simulink model "tcp10"  (R2014a)
settings: Solver=FixedStepDiscrete  StartTime=0.0  StopTime=inf  FixedStep=0.2  RelTol=1e-3
libraries: simulink x6, instrumentlib x4, hdlsllib x2
settings Model: Creator=laca  LastModifiedBy=laca
settings DataIOCC: SignalLoggingSaveFormat=ModelDataLogs

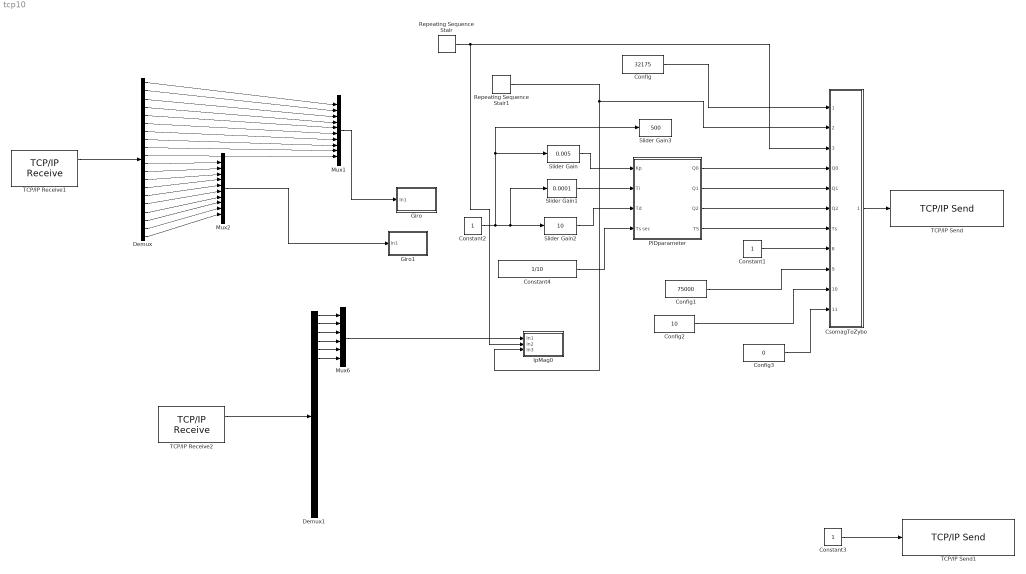
== system tcp10 ==
  Config : Constant  Value=32175
  Config1 : Constant  Value=75000
  Config2 : Constant  Value=10
  Config3 : Constant  Value=0
  Constant1 : Constant
  Constant2 : Constant
  Constant3 : Constant
  Constant4 : Constant  Value=1/10
  CsomagToZybo : Subsystem
  Demux : Demux  Outputs=20
  Demux1 : Demux  Outputs=24
  Giro : Subsystem
  Giro1 : Subsystem
  IpMag0 : Subsystem
  Mux1 : Mux  Inputs=10
  Mux2 : Mux  Inputs=10
  Mux6 : Mux  Inputs=6
  PIDparameter : Subsystem
  Repeating Sequence Stair : simulink/Sources/Repeating Sequence Stair  OutValues=[250*ones(1,1000) 500*ones(1,1000) 800*ones(1,1000) 50*ones(1,1000)].'  tsamp=-1  OutMin=[]  OutMax=[]  OutDataTypeStr=double  OutputDataTypeScalingMode=double  OutDataType=fixdt(0,8)  ConRadixGroup=Best Precision: Vector-wise  OutScaling=2^-12
  Repeating Sequence Stair1 : simulink/Sources/Repeating Sequence Stair  OutValues=[0*ones(1,500) 100*ones(1,500) 77*ones(1,500) -77*ones(1,500) ].'  tsamp=-1  OutMin=[]  OutMax=[]  OutDataTypeStr=double  OutputDataTypeScalingMode=double  OutDataType=fixdt(0,8)  ConRadixGroup=Best Precision: Vector-wise  OutScaling=2^-12
  Slider Gain : simulink/Math Operations/Slider Gain  low=0  gain=0.005  high=65000
  Slider Gain1 : simulink/Math Operations/Slider Gain  low=0  gain=0.0001  high=100000
  Slider Gain2 : simulink/Math Operations/Slider Gain  low=0  gain=10  high=5000
  Slider Gain3 : simulink/Math Operations/Slider Gain  low=-7000  gain=500  high=7000
  TCP/IP Receive1 : instrumentlib/TCP//IP Receive  Host=192.168.0.10  Port=7  DataSize="[1  20]"  EnableBlockingMode=off  Timeout=100  SampleTime=0.2  DataType=int16  ByteOrder=LittleEndian
  TCP/IP Receive2 : instrumentlib/TCP//IP Receive  Host=192.168.0.10  Port=8  DataSize="[1  24]"  EnableBlockingMode=off  Timeout=100  SampleTime=0.2  DataType=int32  ByteOrder=LittleEndian
  TCP/IP Send : instrumentlib/TCP//IP Send  Host=192.168.0.10  Port=7  EnableBlockingMode=off  Timeout=10  ByteOrder=LittleEndian
  TCP/IP Send1 : instrumentlib/TCP//IP Send  Host=192.168.0.10  Port=8  EnableBlockingMode=off  Timeout=10  ByteOrder=LittleEndian
  wires:
  Demux/1 -> Mux1/1
  Demux/2 -> Mux1/2
  Demux/3 -> Mux1/3
  TCP/IP Receive1/1 -> Demux/1
  Mux6/1 -> IpMag0/1(In1)
  Demux/10 -> Mux1/10
  Demux/9 -> Mux1/9
  Demux/8 -> Mux1/8
  Demux/7 -> Mux1/7
  Demux/6 -> Mux1/6
  Demux/5 -> Mux1/5
  Demux/4 -> Mux1/4
  Mux1/1 -> Giro/1(In1)
  CsomagToZybo/1(Out1) -> TCP/IP Send/1
  Constant2/1 -> Slider Gain3/1, Slider Gain/1, Slider Gain1/1, Slider Gain2/1
  Slider Gain/1 -> PIDparameter/1(Kp)
  Slider Gain1/1 -> PIDparameter/2(Ti)
  Slider Gain2/1 -> PIDparameter/3(Td)
  Constant4/1 -> PIDparameter/4(Ts sec)
  PIDparameter/4(TS) -> CsomagToZybo/7(Ts)
  PIDparameter/3(Q2) -> CsomagToZybo/6(Q2)
  PIDparameter/2(Q1) -> CsomagToZybo/5(Q1)
  PIDparameter/1(Q0) -> CsomagToZybo/4(Q0)
  Config/1 -> CsomagToZybo/1(Config)
  Constant1/1 -> CsomagToZybo/8(Egyeb)
  Config1/1 -> CsomagToZybo/9(PwmFrek)
  Config2/1 -> CsomagToZybo/10(qSav)
  Config3/1 -> CsomagToZybo/11(SugaeakAranya)
  Demux/11 -> Mux2/1
  Demux/12 -> Mux2/2
  Demux/13 -> Mux2/3
  Demux/14 -> Mux2/4
  Demux/15 -> Mux2/5
  Demux/16 -> Mux2/6
  Demux/17 -> Mux2/7
  Demux/18 -> Mux2/8
  Demux/19 -> Mux2/9
  Demux/20 -> Mux2/10
  Mux2/1 -> Giro1/1(In1)
  TCP/IP Receive2/1 -> Demux1/1
  Constant3/1 -> TCP/IP Send1/1
  Repeating Sequence Stair/1 -> IpMag0/2(In2), CsomagToZybo/3(RefSpeed)
  Repeating Sequence Stair1/1 -> IpMag0/3(In3), CsomagToZybo/2(RefPos)
  Demux1/6 -> Mux6/6
  Demux1/5 -> Mux6/5
  Demux1/4 -> Mux6/4
  Demux1/3 -> Mux6/3
  Demux1/2 -> Mux6/2
  Demux1/1 -> Mux6/1

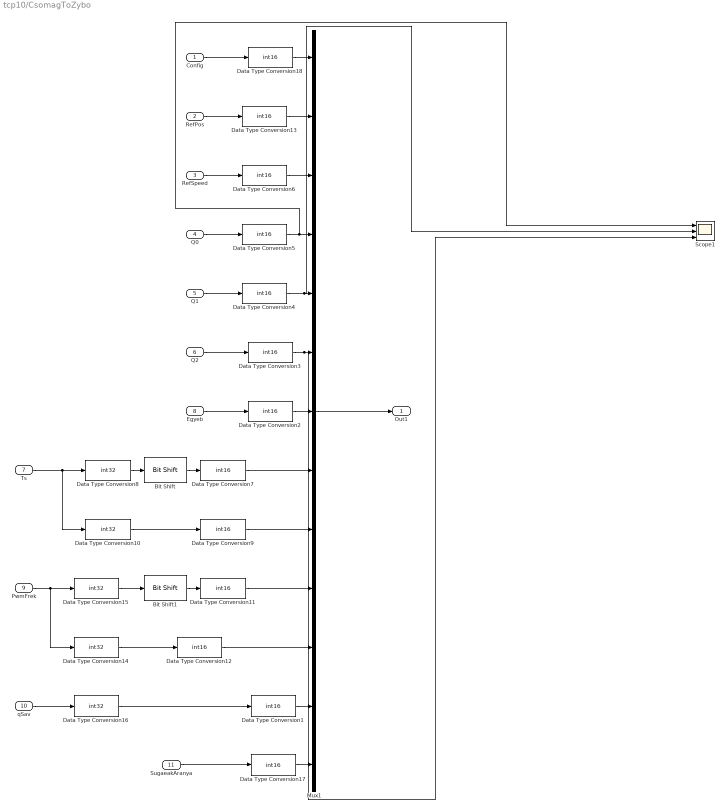
== system tcp10/CsomagToZybo ==
  Config : Inport
  RefPos : Inport  Port=2
  RefSpeed : Inport  Port=3
  Q0 : Inport  Port=4
  Q1 : Inport  Port=5
  Q2 : Inport  Port=6
  Ts : Inport  Port=7
  Egyeb : Inport  Port=8
  PwmFrek : Inport  Port=9
  qSav : Inport  Port=10
  SugaeakAranya : Inport  Port=11
  Bit Shift : hdlsllib/HDL Operations/Bit Shift  mode=Shift Right Arithmetic  N=16
  Bit Shift1 : hdlsllib/HDL Operations/Bit Shift  mode=Shift Right Arithmetic  N=16
  Data Type Conversion{1..7,9,11..13,17..18} (13 alike) : DataTypeConversion  OutDataTypeStr=int16
  Data Type Conversion{8,10,14..16} (5 alike) : DataTypeConversion  OutDataTypeStr=int32
  Mux1 : Mux  Inputs=13
  Scope1 : Scope  NumInputPorts=3
      settings: YMin=1425~-525~-1  YMax=1575~-475~1  SaveName=ScopeData5
  Out1 : Outport
  wires:
  Mux1/1 -> Out1/1
  Data Type Conversion18/1 -> Mux1/1
  Data Type Conversion13/1 -> Mux1/2
  Data Type Conversion6/1 -> Mux1/3
  Data Type Conversion2/1 -> Mux1/7
  Config/1 -> Data Type Conversion18/1
  RefPos/1 -> Data Type Conversion13/1
  RefSpeed/1 -> Data Type Conversion6/1
  Q0/1 -> Data Type Conversion5/1
  Q1/1 -> Data Type Conversion4/1
  Q2/1 -> Data Type Conversion3/1
  Egyeb/1 -> Data Type Conversion2/1
  Ts/1 -> Data Type Conversion10/1, Data Type Conversion8/1
  Data Type Conversion10/1 -> Data Type Conversion9/1
  Data Type Conversion8/1 -> Bit Shift/1
  Bit Shift/1 -> Data Type Conversion7/1
  Data Type Conversion1/1 -> Mux1/12
  PwmFrek/1 -> Data Type Conversion14/1, Data Type Conversion15/1
  Data Type Conversion14/1 -> Data Type Conversion12/1
  Data Type Conversion15/1 -> Bit Shift1/1
  Bit Shift1/1 -> Data Type Conversion11/1
  Data Type Conversion16/1 -> Data Type Conversion1/1
  qSav/1 -> Data Type Conversion16/1
  Data Type Conversion17/1 -> Mux1/13
  SugaeakAranya/1 -> Data Type Conversion17/1
  Data Type Conversion7/1 -> Mux1/8
  Data Type Conversion9/1 -> Mux1/9
  Data Type Conversion11/1 -> Mux1/10
  Data Type Conversion12/1 -> Mux1/11
  Data Type Conversion5/1 -> Scope1/1, Mux1/4
  Data Type Conversion4/1 -> Scope1/2, Mux1/5
  Data Type Conversion3/1 -> Scope1/3, Mux1/6

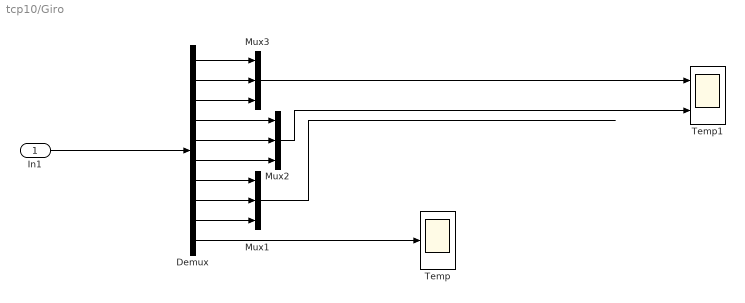
== system tcp10/Giro ==
  In1 : Inport
  Demux : Demux  Outputs=10
  Mux1 : Mux  Inputs=3
  Mux2 : Mux  Inputs=3
  Mux3 : Mux  Inputs=3
  Temp : Scope
      settings: TickLabels=on  TimeRange=2000  YMin=204.25  YMax=225.75  SaveName=ScopeData4  SampleInput=on
  Temp1 : Scope  NumInputPorts=2
      settings: TickLabels=on  TimeRange=250  YMin=-35000~-35000  YMax=35000~35000  SaveName=ScopeData2  SampleInput=on
  wires:
  In1/1 -> Demux/1
  Demux/1 -> Mux3/1
  Demux/2 -> Mux3/2
  Demux/3 -> Mux3/3
  Demux/4 -> Mux2/1
  Demux/5 -> Mux2/2
  Demux/6 -> Mux2/3
  Demux/7 -> Mux1/1
  Demux/8 -> Mux1/2
  Demux/9 -> Mux1/3
  Mux3/1 -> Temp1/1
  Mux2/1 -> Temp1/2
  Mux1/1 -> ?
  Demux/10 -> Temp/1

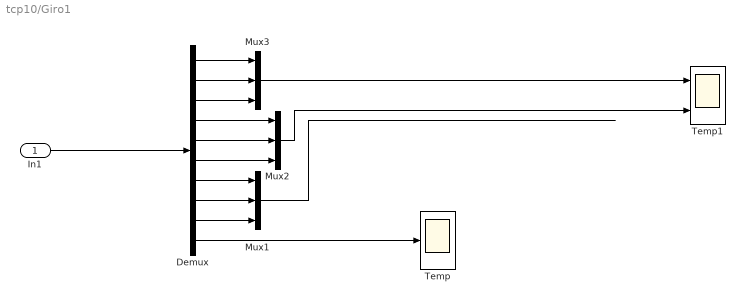
== system tcp10/Giro1 ==
  In1 : Inport
  Demux : Demux  Outputs=10
  Mux1 : Mux  Inputs=3
  Mux2 : Mux  Inputs=3
  Mux3 : Mux  Inputs=3
  Temp : Scope
      settings: TickLabels=on  TimeRange=2000  YMin=36  YMax=36  SaveName=ScopeData4  SampleInput=on
  Temp1 : Scope  NumInputPorts=2
      settings: TickLabels=on  TimeRange=250  YMin=-65500~-35000  YMax=65500~35000  SaveName=ScopeData2  SampleInput=on
  wires:
  In1/1 -> Demux/1
  Demux/1 -> Mux3/1
  Demux/2 -> Mux3/2
  Demux/3 -> Mux3/3
  Demux/4 -> Mux2/1
  Demux/5 -> Mux2/2
  Demux/6 -> Mux2/3
  Demux/7 -> Mux1/1
  Demux/8 -> Mux1/2
  Demux/9 -> Mux1/3
  Mux3/1 -> Temp1/1
  Mux2/1 -> Temp1/2
  Mux1/1 -> ?
  Demux/10 -> Temp/1

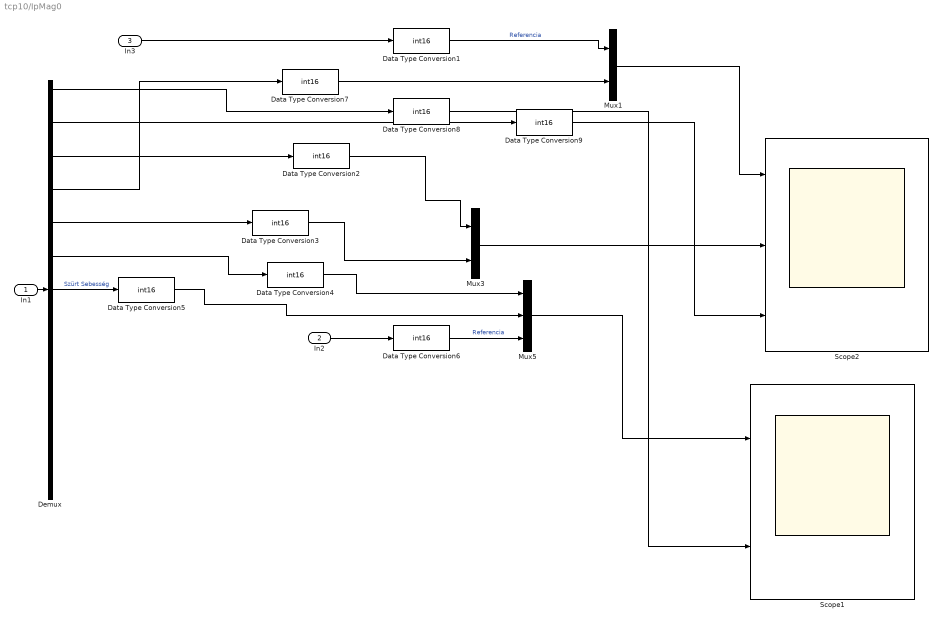
== system tcp10/IpMag0 ==
  In1 : Inport
  In2 : Inport  Port=2
  In3 : Inport  Port=3
  Data Type Conversion{1..9} (9 alike) : DataTypeConversion  OutDataTypeStr=int16
  Demux : Demux  Outputs=13
  Mux1 : Mux  Inputs=2
  Mux3 : Mux  Inputs=2
  Mux5 : Mux  Inputs=3
  Scope1 : Scope  NumInputPorts=2
      settings: TickLabels=on  TimeRange=2000  YMin=0~-35000  YMax=800~35000  SampleInput=on
  Scope2 : Scope  NumInputPorts=3
      settings: TickLabels=on  TimeRange=500  YMin=-250~-60~-562.8  YMax=4750~70~-509.2  SaveName=ScopeData3  SampleInput=on
  wires:
  Demux/3 -> Data Type Conversion2/1
  Demux/5 -> Data Type Conversion3/1
  Demux/6 -> Data Type Conversion4/1
  Demux/7 -> Data Type Conversion5/1  "Szürt Sebesség"
  Mux3/1 -> Scope2/2
  In1/1 -> Demux/1
  Mux5/1 -> Scope1/1
  In2/1 -> Data Type Conversion6/1
  Demux/1 -> Data Type Conversion8/1
  Demux/2 -> Data Type Conversion9/1
  Data Type Conversion6/1 -> Mux5/3  "Referencia"
  In3/1 -> Data Type Conversion1/1
  Demux/4 -> Data Type Conversion7/1
  Mux1/1 -> Scope2/1
  Data Type Conversion1/1 -> Mux1/1  "Referencia"
  Data Type Conversion2/1 -> Mux3/1
  Data Type Conversion3/1 -> Mux3/2
  Data Type Conversion4/1 -> Mux5/1
  Data Type Conversion5/1 -> Mux5/2
  Data Type Conversion7/1 -> Mux1/2
  Data Type Conversion8/1 -> Scope1/2
  Data Type Conversion9/1 -> Scope2/3

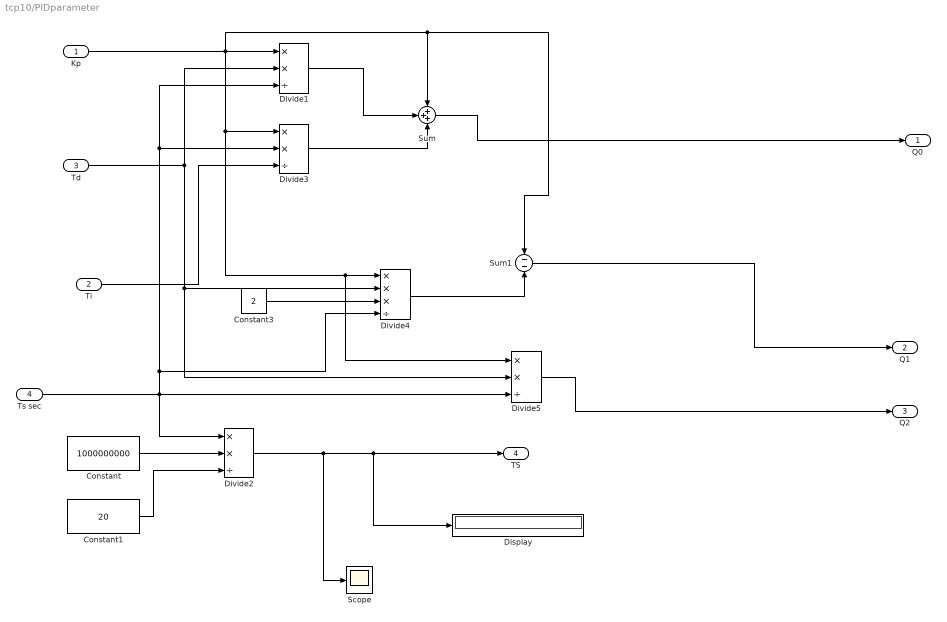
== system tcp10/PIDparameter ==
  Kp : Inport
  Ti : Inport  Port=2
  Td : Inport  Port=3
  Ts sec : Inport  Port=4
  Constant : Constant  Value=1000000000
  Constant1 : Constant  Value=20
  Constant3 : Constant  Value=2
  Display : Display
  Divide{1..3,5} (4 alike) : Product  Inputs=**/
  Divide4 : Product  Inputs=***/
  Scope : Scope
  Sum : Sum  Inputs=+++
  Sum1 : Sum  Inputs=--
  Q0 : Outport
  Q1 : Outport  Port=2
  Q2 : Outport  Port=3
  TS : Outport  Port=4
  wires:
  Divide2/1 -> Scope/1, Display/1, TS/1
  Ts sec/1 -> Divide5/3, Divide2/1, Divide4/4, Divide3/2, Divide1/3
  Constant/1 -> Divide2/2
  Constant1/1 -> Divide2/3
  Ti/1 -> Divide3/3
  Td/1 -> Divide1/2, Divide5/2, Divide4/2
  Divide3/1 -> Sum/3
  Divide1/1 -> Sum/2
  Kp/1 -> Sum1/1, Sum/1, Divide5/1, Divide4/1, Divide3/1, Divide1/1
  Constant3/1 -> Divide4/3
  Divide4/1 -> Sum1/2
  Sum/1 -> Q0/1
  Sum1/1 -> Q1/1
  Divide5/1 -> Q2/1
